simulink model "Admittance"  (R2022b)
settings: Solver=VariableStepAuto  StartTime=0.0  StopTime=10.0  RelTol=1e-3
values from neighbouring files (symbols this model uses):
  Kd = diag([10,10,10,1,1,1])    [parameters.m]
  Kdt = diag([5,5,5,1,1,1])    [parameters.m]
  Kp = diag([190,190,190,1,1,1])    [parameters.m]
  Kpt = diag([50,50,50,1,1,1])    [parameters.m]
  Md = diag([0.12,0.12,0.12,0,0,0])    [parameters.m]
  Mt = diag([1,1,1,1,1,1])    [parameters.m]
undefined symbols (not defined in the file or in its folder): parms
libraries: robotcorelib x1
settings Model: Creator=uzair  LastModifiedBy=uzair

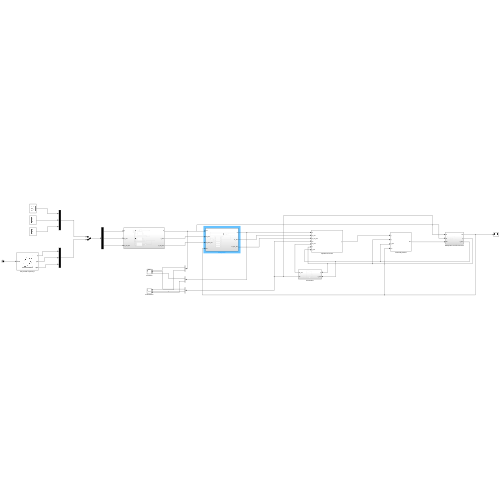
[thumbnail: Simulink's stored preview of the top-level diagram]
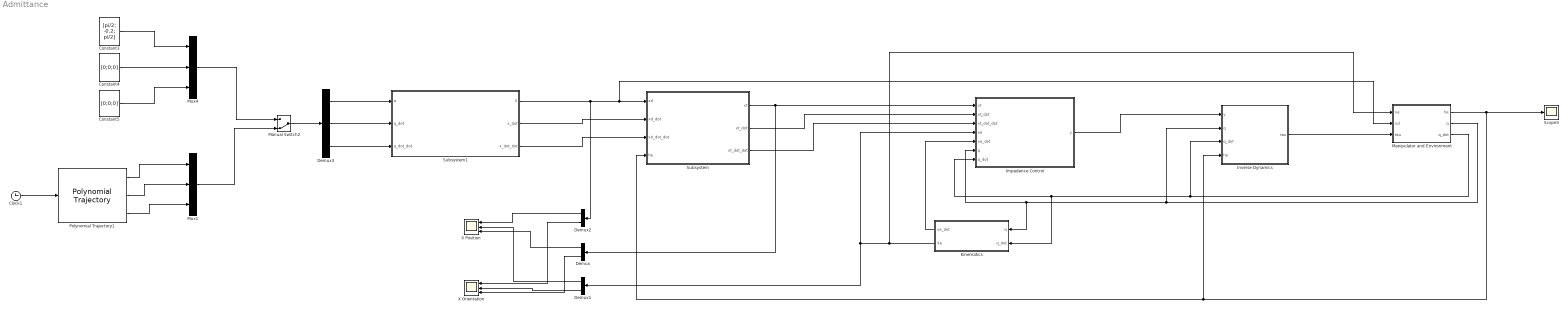
== system Admittance ==
  Clock1 : Clock
  Constant3 : Constant  Value=[pi/2; -0.2; pi/2]  VectorParams1D=off
  Constant4 : Constant  Value=[0;0;0]  VectorParams1D=off
  Constant5 : Constant  Value=[0;0;0]  VectorParams1D=off
  Demux : Demux  Outputs=2
  Demux1 : Demux  Outputs=2
  Demux2 : Demux  Outputs=2
  Demux3 : Demux  Outputs=3
  Impedence Control : Subsystem
  Inverse Dynamics : Subsystem
  Kinematics : Subsystem
  Manipulator and Environment : Subsystem
  Manual Switch2 : ManualSwitch  CurrentSetting=0
  Mux1 : Mux  Inputs=3
  Mux4 : Mux  Inputs=3
  Polynomial Trajectory1 : robotcorelib/Polynomial Trajectory  WaypointSource=Internal  Waypoints=[ 0,0.5,0.7,0.9; 0,-0.05,-0.1,-0.15; 0,0.5,0.7,0.9]  TimePoints=[ 0, 4, 7, 10]  TimeInterval=[ 1, 4 ]  Method=Quintic Polynomial  ParameterSource=Internal  VelocityBoundaryCondition=zeros( 3,4 )  AccelerationBoundaryCondition=zeros( 3,4 )  SimulateUsing=Interpreted execution
  Scope3 : Scope
  Subsystem : Subsystem
  Subsystem1 : Subsystem
  X Orientation : Scope  NumInputPorts=3
  X Position : Scope  NumInputPorts=3
  wires:
  Demux1/2 -> X Orientation/2
  Demux2/2 -> X Orientation/1
  Demux2/1 -> X Position/1
  Demux1/1 -> X Position/2
  Manual Switch2/1 -> Demux3/1
  Mux4/1 -> Manual Switch2/1
  Constant4/1 -> Mux4/2
  Polynomial Trajectory1/1 -> Mux1/1
  Polynomial Trajectory1/3 -> Mux1/3
  Mux1/1 -> Manual Switch2/2
  Constant5/1 -> Mux4/3
  Clock1/1 -> Polynomial Trajectory1/1
  Constant3/1 -> Mux4/1
  Demux3/3 -> Subsystem1/3(q_dot_dot)
  Polynomial Trajectory1/2 -> Mux1/2
  Demux3/2 -> Subsystem1/2(q_dot)
  Impedence Control/1(y) -> Inverse Dynamics/1(y)
  Kinematics/2(Xe) -> Manipulator and Environment/1(xe), Demux1/1, Impedence Control/4(xe)
  Kinematics/1(xe_dot) -> Impedence Control/5(xe_dot)
  Manipulator and Environment/2(q) -> Inverse Dynamics/2(q), Kinematics/1(q), Impedence Control/6(q)
  Manipulator and Environment/3(q_dot) -> Inverse Dynamics/3(q_dot), Kinematics/2(q_dot), Impedence Control/7(q_dot)
  Manipulator and Environment/1(he) -> Scope3/1, Inverse Dynamics/4(he), Subsystem/4(he)
  Inverse Dynamics/1(tau) -> Manipulator and Environment/3(tau)
  Demux3/1 -> Subsystem1/1(q)
  Subsystem1/1(X) -> Demux2/1, Manipulator and Environment/2(xd), Subsystem/1(xd)
  Subsystem1/2(x_dot) -> Subsystem/2(xd_dot)
  Subsystem1/3(x_dot_dot) -> Subsystem/3(xd_dot_dot)
  Subsystem/1(xt) -> Demux/1, Impedence Control/1(xt)
  Subsystem/2(xt_dot) -> Impedence Control/2(xt_dot)
  Subsystem/3(xt_dot_dot) -> Impedence Control/3(xt_dot_dot)
  Demux/1 -> X Position/3
  Demux/2 -> X Orientation/3

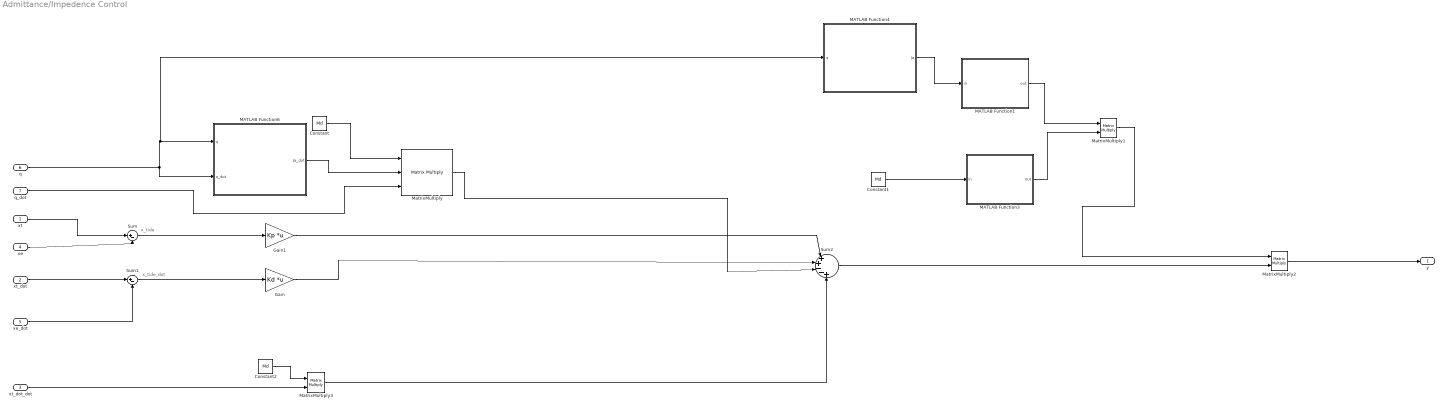
== system Admittance/Impedence Control ==
  note: x_tide_dot
  note: x_tide
  xt : Inport
  xt_dot : Inport  Port=2
  xt_dot_dot : Inport  Port=3
  xe : Inport  Port=4
  xe_dot : Inport  Port=5
  q : Inport  Port=6
  q_dot : Inport  Port=7
  Constant : Constant  Value=Md  VectorParams1D=off
  Constant1 : Constant  Value=Md  VectorParams1D=off
  Constant2 : Constant  Value=Md
  Gain : Gain  Gain=Kd  Multiplication=Matrix(K*u)
  Gain1 : Gain  Gain=Kp  Multiplication=Matrix(K*u)
  MATLAB Function1 : MATLAB Function  TreatAsAtomicUnit=on
  MATLAB Function3 : MATLAB Function  TreatAsAtomicUnit=on
  MATLAB Function4 : MATLAB Function  TreatAsAtomicUnit=on
  MATLAB Function6 : MATLAB Function  TreatAsAtomicUnit=on
  MatrixMultiply : Product  Inputs=3  Multiplication=Matrix(*)
  MatrixMultiply1 : Product  Multiplication=Matrix(*)
  MatrixMultiply2 : Product  Multiplication=Matrix(*)
  MatrixMultiply3 : Product  Multiplication=Matrix(*)
  Sum : Sum  Inputs=|+-
  Sum1 : Sum  Inputs=|+-
  Sum2 : Sum  Inputs=|++--+
  y : Outport
  wires:
  xt/1 -> Sum/1
  xe/1 -> Sum/2
  Sum/1 -> Gain1/1
  xt_dot/1 -> Sum1/1
  xe_dot/1 -> Sum1/2
  Sum1/1 -> Gain/1
  Gain1/1 -> Sum2/1
  Gain/1 -> Sum2/2
  q/1 -> MATLAB Function6/2(q_dot), MATLAB Function4/1(q), MATLAB Function6/1(q)
  q_dot/1 -> MatrixMultiply/3
  Constant/1 -> MatrixMultiply/1
  MATLAB Function6/1(Ja_dot) -> MatrixMultiply/2
  MatrixMultiply/1 -> Sum2/3
  MATLAB Function1/1(out) -> MatrixMultiply1/1
  MATLAB Function3/1(out) -> MatrixMultiply1/2
  MATLAB Function4/1(Ja) -> MATLAB Function1/1(in)
  Constant1/1 -> MATLAB Function3/1(in)
  Sum2/1 -> MatrixMultiply2/2
  MatrixMultiply1/1 -> MatrixMultiply2/1
  MatrixMultiply2/1 -> y/1
  xt_dot_dot/1 -> MatrixMultiply3/2
  Constant2/1 -> MatrixMultiply3/1
  MatrixMultiply3/1 -> Sum2/5

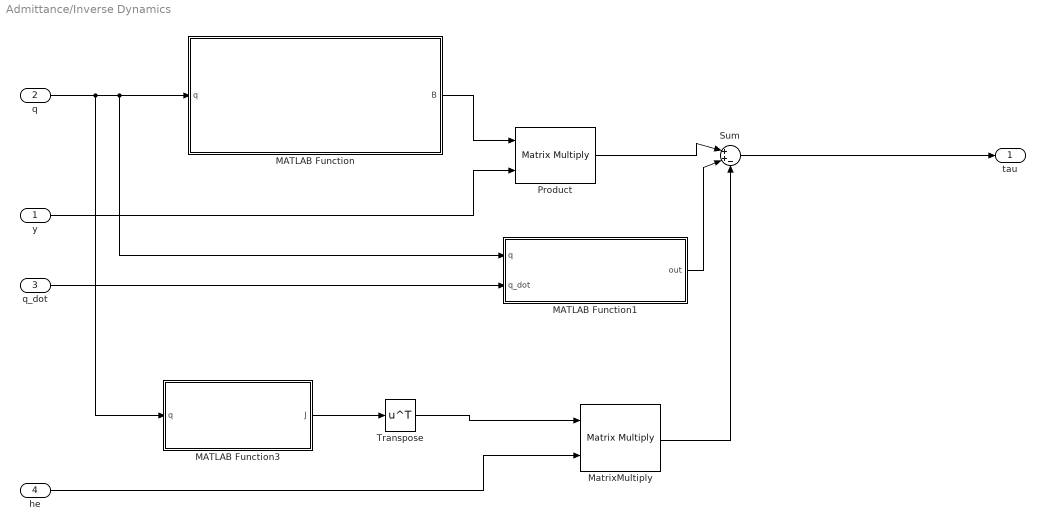
== system Admittance/Inverse Dynamics ==
  y : Inport
  q : Inport  Port=2
  q_dot : Inport  Port=3
  he : Inport  Port=4
  MATLAB Function : MATLAB Function  TreatAsAtomicUnit=on
  MATLAB Function1 : MATLAB Function  TreatAsAtomicUnit=on
  MATLAB Function3 : MATLAB Function  TreatAsAtomicUnit=on
  MatrixMultiply : Product  Multiplication=Matrix(*)
  Product : Product  Multiplication=Matrix(*)
  Sum : Sum  Inputs=|++-
  Transpose : Math  Operator=transpose  OutputSignalType=real
  tau : Outport
  wires:
  q/1 -> MATLAB Function3/1(q), MATLAB Function1/1(q), MATLAB Function/1(q)
  MATLAB Function/1(B) -> Product/1
  y/1 -> Product/2
  q_dot/1 -> MATLAB Function1/2(q_dot)
  MATLAB Function1/1(out) -> Sum/2
  Sum/1 -> tau/1
  MATLAB Function3/1(J) -> Transpose/1
  he/1 -> MatrixMultiply/2
  Transpose/1 -> MatrixMultiply/1
  MatrixMultiply/1 -> Sum/3
  Product/1 -> Sum/1

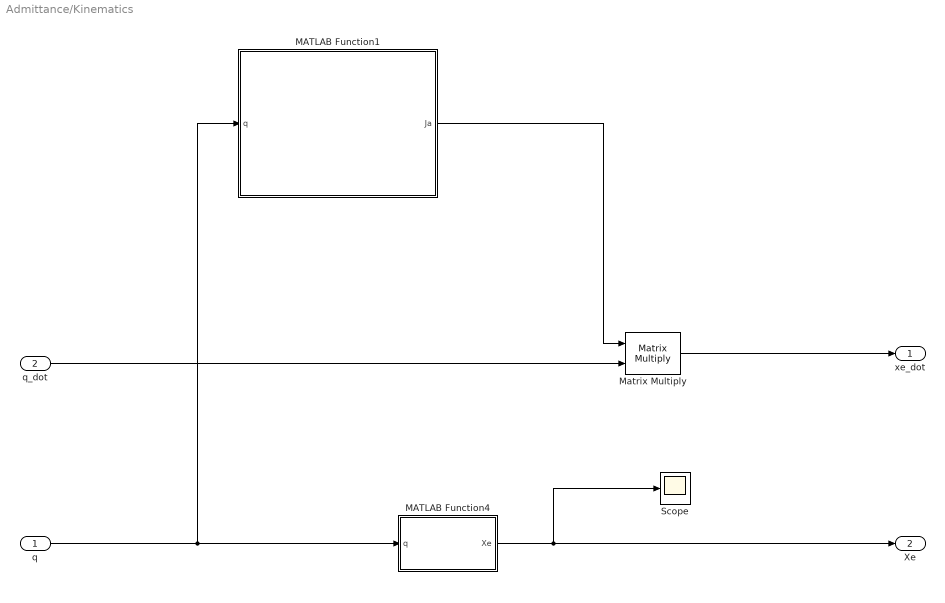
== system Admittance/Kinematics ==
  q : Inport
  q_dot : Inport  Port=2
  MATLAB Function1 : MATLAB Function  TreatAsAtomicUnit=on
  MATLAB Function4 : MATLAB Function  TreatAsAtomicUnit=on
  Matrix Multiply : Product  Multiplication=Matrix(*)
  Scope : Scope
  xe_dot : Outport
  Xe : Outport  Port=2
  wires:
  MATLAB Function1/1(Ja) -> Matrix Multiply/1
  q/1 -> MATLAB Function1/1(q), MATLAB Function4/1(q)
  MATLAB Function4/1(Xe) -> Scope/1, Xe/1
  Matrix Multiply/1 -> xe_dot/1
  q_dot/1 -> Matrix Multiply/2

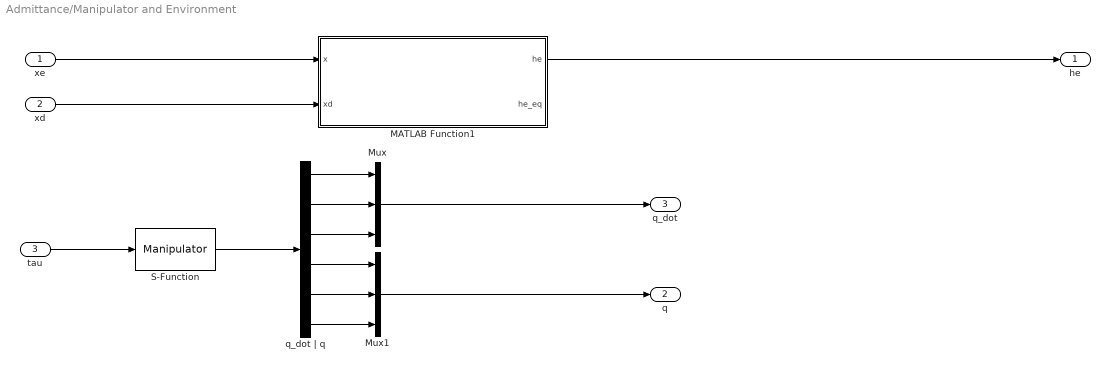
== system Admittance/Manipulator and Environment ==
  xe : Inport
  xd : Inport  Port=2
  tau : Inport  Port=3
  MATLAB Function1 : MATLAB Function  TreatAsAtomicUnit=on
  Mux : Mux  Inputs=3
  Mux1 : Mux  Inputs=3
  S-Function : S-Function  FunctionName=Manipulator  Parameters=params  SFunctionDeploymentMode=off  EnableBusSupport=off
  q_dot | q : Demux  Outputs=6
  he : Outport
  q : Outport  Port=2
  q_dot : Outport  Port=3
  wires:
  xe/1 -> MATLAB Function1/1(x)
  xd/1 -> MATLAB Function1/2(xd)
  MATLAB Function1/1(he) -> he/1
  S-Function/1 -> q_dot | q/1
  q_dot | q/4 -> Mux1/1
  q_dot | q/1 -> Mux/1
  q_dot | q/6 -> Mux1/3
  q_dot | q/2 -> Mux/2
  q_dot | q/5 -> Mux1/2
  q_dot | q/3 -> Mux/3
  Mux/1 -> q_dot/1
  Mux1/1 -> q/1
  tau/1 -> S-Function/1

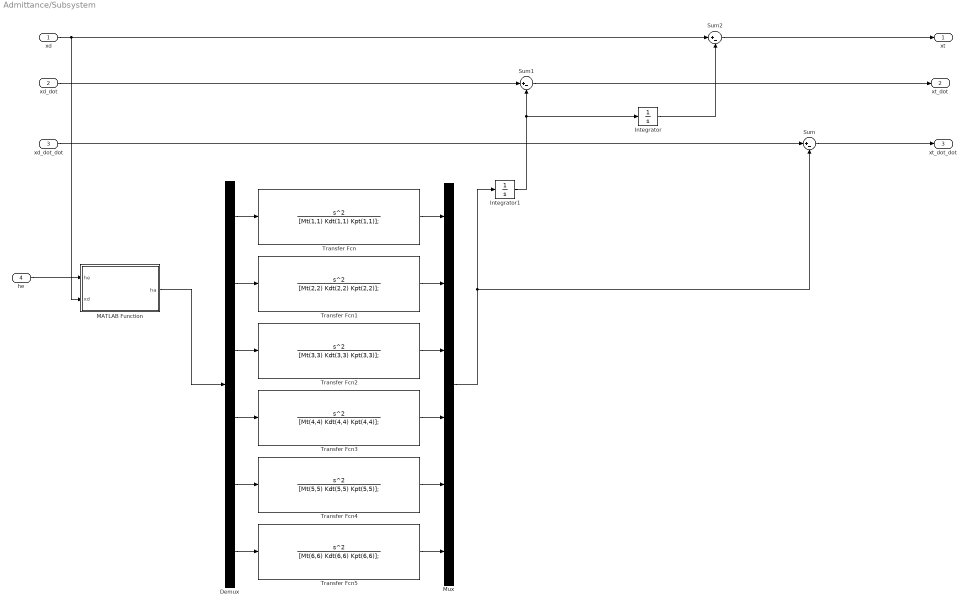
== system Admittance/Subsystem ==
  xd : Inport
  xd_dot : Inport  Port=2
  xd_dot_dot : Inport  Port=3
  he : Inport  Port=4
  Demux : Demux  Outputs=6
  Integrator : Integrator
  Integrator1 : Integrator
  MATLAB Function : MATLAB Function  TreatAsAtomicUnit=on
  Mux : Mux  Inputs=6
  Sum : Sum  Inputs=|+-
  Sum1 : Sum  Inputs=|+-
  Sum2 : Sum  Inputs=|+-
  Transfer Fcn : TransferFcn  Numerator=[1 0 0]  Denominator=[Mt(1,1) Kdt(1,1) Kpt(1,1)];
  Transfer Fcn1 : TransferFcn  Numerator=[1 0 0]  Denominator=[Mt(2,2) Kdt(2,2) Kpt(2,2)];
  Transfer Fcn2 : TransferFcn  Numerator=[1 0 0]  Denominator=[Mt(3,3) Kdt(3,3) Kpt(3,3)];
  Transfer Fcn3 : TransferFcn  Numerator=[1 0 0]  Denominator=[Mt(4,4) Kdt(4,4) Kpt(4,4)];
  Transfer Fcn4 : TransferFcn  Numerator=[1 0 0]  Denominator=[Mt(5,5) Kdt(5,5) Kpt(5,5)];
  Transfer Fcn5 : TransferFcn  Numerator=[1 0 0]  Denominator=[Mt(6,6) Kdt(6,6) Kpt(6,6)];
  xt : Outport
  xt_dot : Outport  Port=2
  xt_dot_dot : Outport  Port=3
  wires:
  he/1 -> MATLAB Function/1(he)
  xd/1 -> Sum2/1, MATLAB Function/2(xd)
  Sum2/1 -> xt/1
  xd_dot/1 -> Sum1/1
  Sum1/1 -> xt_dot/1
  Sum/1 -> xt_dot_dot/1
  xd_dot_dot/1 -> Sum/1
  MATLAB Function/1(ha) -> Demux/1
  Mux/1 -> Integrator1/1, Sum/2
  Integrator1/1 -> Integrator/1, Sum1/2
  Integrator/1 -> Sum2/2
  Transfer Fcn/1 -> Mux/1
  Demux/1 -> Transfer Fcn/1
  Demux/2 -> Transfer Fcn1/1
  Transfer Fcn1/1 -> Mux/2
  Demux/3 -> Transfer Fcn2/1
  Transfer Fcn2/1 -> Mux/3
  Transfer Fcn3/1 -> Mux/4
  Demux/4 -> Transfer Fcn3/1
  Transfer Fcn4/1 -> Mux/5
  Demux/5 -> Transfer Fcn4/1
  Transfer Fcn5/1 -> Mux/6
  Demux/6 -> Transfer Fcn5/1

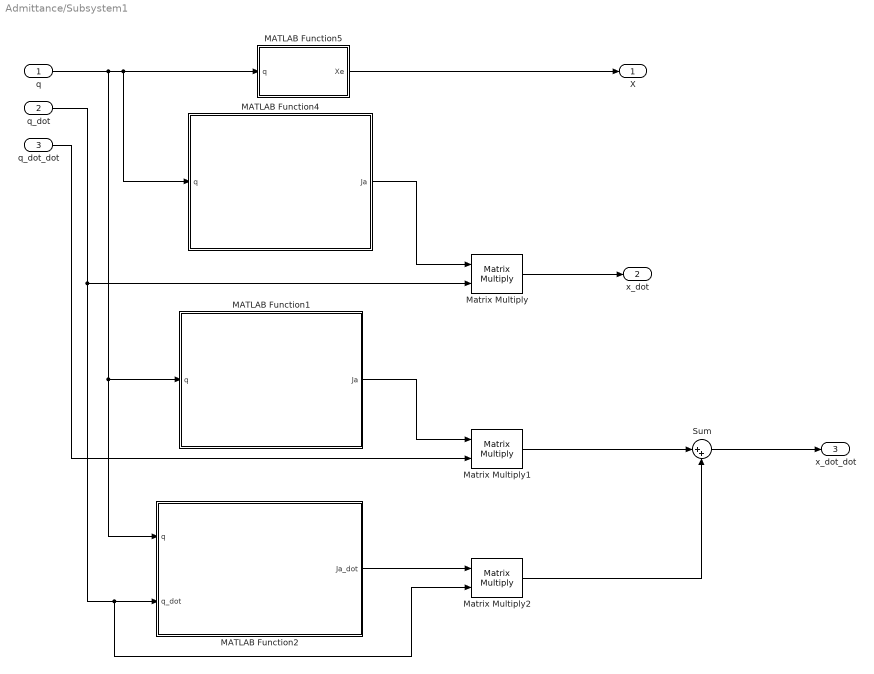
== system Admittance/Subsystem1 ==
  q : Inport
  q_dot : Inport  Port=2
  q_dot_dot : Inport  Port=3
  MATLAB Function1 : MATLAB Function  TreatAsAtomicUnit=on
  MATLAB Function2 : MATLAB Function  TreatAsAtomicUnit=on
  MATLAB Function4 : MATLAB Function  TreatAsAtomicUnit=on
  MATLAB Function5 : MATLAB Function  TreatAsAtomicUnit=on
  Matrix Multiply : Product  Multiplication=Matrix(*)
  Matrix Multiply1 : Product  Multiplication=Matrix(*)  SaturateOnIntegerOverflow=on  LockScale=on
  Matrix Multiply2 : Product  Multiplication=Matrix(*)  InputSameDT=on  SaturateOnIntegerOverflow=on
  Sum : Sum  Inputs=|++
  X : Outport
  x_dot : Outport  Port=2
  x_dot_dot : Outport  Port=3
  wires:
  q/1 -> MATLAB Function2/1(q), MATLAB Function1/1(q), MATLAB Function4/1(q), MATLAB Function5/1(q)
  MATLAB Function5/1(Xe) -> X/1
  Matrix Multiply/1 -> x_dot/1
  q_dot/1 -> MATLAB Function2/2(q_dot), Matrix Multiply2/2, Matrix Multiply/2
  MATLAB Function4/1(Ja) -> Matrix Multiply/1
  MATLAB Function1/1(Ja) -> Matrix Multiply1/1
  q_dot_dot/1 -> Matrix Multiply1/2
  Matrix Multiply1/1 -> Sum/1
  Sum/1 -> x_dot_dot/1
  MATLAB Function2/1(Ja_dot) -> Matrix Multiply2/1
  Matrix Multiply2/1 -> Sum/2

== matlab function Admittance/Impedence Control/MATLAB Function6 ==
  data: q input; Ja_dot output; q_dot input
function Ja_dot = AnalyticalJacobian_Dot(q, q_dot)
q1 = q(1);
q2 = q(2);
q3 = q(3);

q1_dot = q_dot(1);
q2_dot = q_dot(2);
q3_dot = q_dot(3);

H = [[       0,         -cos(q3),        -sin(q3),                                                     -(4*sin(q3))/25]
[ sin(q1), -cos(q1)*sin(q3), cos(q1)*cos(q3),        (2*cos(q1))/5 + (4*cos(q1)*cos(q3))/25 - sin(q1)*(q2 + 3/10)]
[-cos(q1), -sin(q1)*sin(q3), cos(q3)*sin(q1), (2*sin(q1))/5 + cos(q1)*(q2 + 3/10) + (4*cos(q3)*sin(q1))/25 + 3/20]
[       0,                0,               0,                                                                   1]];



eulers = rotm2eul(H(1:3,1:3), "ZYZ");


phi1 = eulers(1);
phi2 = eulers(2);
phi3 = eulers(3); %not used

Ja_dot_m = [
[                                                                                                                                   0,               0,                                                 (4*q3_dot*sin(q3))/25]
[  q1_dot*sin(q1)*(q2 + 3/10) - q2_dot*cos(q1) - (4*q1_dot*cos(q1)*cos(q3))/25 - (2*q1_dot*cos(q1))/5 + (4*q3_dot*sin(q1)*sin(q3))/25, -q1_dot*cos(q1),         (4*q1_dot*sin(q1)*sin(q3))/25 - (4*q3_dot*cos(q1)*cos(q3))/25]
[- (2*q1_dot*sin(q1))/5 - q2_dot*sin(q1) - q1_dot*cos(q1)*(q2 + 3/10) - (4*q1_dot*cos(q3)*sin(q1))/25 - (4*q3_dot*cos(q1)*sin(q3))/25, -q1_dot*sin(q1),       - (4*q1_dot*cos(q1)*sin(q3))/25 - (4*q3_dot*cos(q3)*sin(q1))/25]
[                                                                                                                                   0,               0, -(q1_dot*(sin(phi2)*sin(q1) - cos(phi2)*cos(q1)*sin(phi1)))/sin(phi2)]
[                                                                                                                                   0,               0,                                             -q1_dot*cos(phi1)*cos(q1)]
[                                                                                                                                   0,               0,                                 -(q1_dot*cos(q1)*sin(phi1))/sin(phi2)]
];

Ja_dot = Ja_dot_m;
end

== matlab function Admittance/Subsystem1/MATLAB Function2 ==
  data: q input; Ja_dot output; q_dot input
function Ja_dot = AnalyticalJacobian_Dot(q, q_dot)
q1 = q(1);
q2 = q(2);
q3 = q(3);

q1_dot = q_dot(1);
q2_dot = q_dot(2);
q3_dot = q_dot(3);

H = [[       0,         -cos(q3),        -sin(q3),                                                     -(4*sin(q3))/25]
[ sin(q1), -cos(q1)*sin(q3), cos(q1)*cos(q3),        (2*cos(q1))/5 + (4*cos(q1)*cos(q3))/25 - sin(q1)*(q2 + 3/10)]
[-cos(q1), -sin(q1)*sin(q3), cos(q3)*sin(q1), (2*sin(q1))/5 + cos(q1)*(q2 + 3/10) + (4*cos(q3)*sin(q1))/25 + 3/20]
[       0,                0,               0,                                                                   1]];



eulers = rotm2eul(H(1:3,1:3), "ZYZ");


phi1 = eulers(1);
phi2 = eulers(2);
phi3 = eulers(3); %not used

Ja_dot_m = [
[                                                                                                                                   0,               0,                                                 (4*q3_dot*sin(q3))/25]
[  q1_dot*sin(q1)*(q2 + 3/10) - q2_dot*cos(q1) - (4*q1_dot*cos(q1)*cos(q3))/25 - (2*q1_dot*cos(q1))/5 + (4*q3_dot*sin(q1)*sin(q3))/25, -q1_dot*cos(q1),         (4*q1_dot*sin(q1)*sin(q3))/25 - (4*q3_dot*cos(q1)*cos(q3))/25]
[- (2*q1_dot*sin(q1))/5 - q2_dot*sin(q1) - q1_dot*cos(q1)*(q2 + 3/10) - (4*q1_dot*cos(q3)*sin(q1))/25 - (4*q3_dot*cos(q1)*sin(q3))/25, -q1_dot*sin(q1),       - (4*q1_dot*cos(q1)*sin(q3))/25 - (4*q3_dot*cos(q3)*sin(q1))/25]
[                                                                                                                                   0,               0, -(q1_dot*(sin(phi2)*sin(q1) - cos(phi2)*cos(q1)*sin(phi1)))/sin(phi2)]
[                                                                                                                                   0,               0,                                             -q1_dot*cos(phi1)*cos(q1)]
[                                                                                                                                   0,               0,                                 -(q1_dot*cos(q1)*sin(phi1))/sin(phi2)]
];

Ja_dot = Ja_dot_m;
end

== matlab function Admittance/Subsystem1/MATLAB Function4 ==
  data: q input; Ja output
function Ja = AnalyticalJacobian(q)
    q1 = q(1);
    q2 = q(2);
    q3 = q(3);

    H = [[       0,         -cos(q3),        -sin(q3),                                                     -(4*sin(q3))/25]
[ sin(q1), -cos(q1)*sin(q3), cos(q1)*cos(q3),        (2*cos(q1))/5 + (4*cos(q1)*cos(q3))/25 - sin(q1)*(q2 + 3/10)]
[-cos(q1), -sin(q1)*sin(q3), cos(q3)*sin(q1), (2*sin(q1))/5 + cos(q1)*(q2 + 3/10) + (4*cos(q3)*sin(q1))/25 + 3/20]
[       0,                0,               0,                                                                   1]];


eulers = rotm2eul(H(1:3,1:3), "ZYZ");


    phi1 = eulers(1);
    phi2 = eulers(2);
    phi3 = eulers(3); %not used

Ja_m = [
[                                                             0,        0,                                             -(4*cos(q3))/25]
[- (2*sin(q1))/5 - cos(q1)*(q2 + 3/10) - (4*cos(q3)*sin(q1))/25, -sin(q1),                                     -(4*cos(q1)*sin(q3))/25]
[  (2*cos(q1))/5 + (4*cos(q1)*cos(q3))/25 - sin(q1)*(q2 + 3/10),  cos(q1),                                     -(4*sin(q1)*sin(q3))/25]
[                              -(cos(phi1)*cos(phi2))/sin(phi2),        0, (cos(q1)*sin(phi2) + cos(phi2)*sin(phi1)*sin(q1))/sin(phi2)]
[                                                    -sin(phi1),        0,                                          -cos(phi1)*sin(q1)]
[                                           cos(phi1)/sin(phi2),        0,                              -(sin(phi1)*sin(q1))/sin(phi2)]
];


    Ja = Ja_m;
end

== matlab function Admittance/Subsystem1/MATLAB Function5 ==
  data: q input; Xe output
function Xe = Kinematics(q)
    q1 = q(1);
    q2 = q(2);
    q3 = q(3);
    
H = [[       0,         -cos(q3),        -sin(q3),                                                     -(4*sin(q3))/25]
[ sin(q1), -cos(q1)*sin(q3), cos(q1)*cos(q3),        (2*cos(q1))/5 + (4*cos(q1)*cos(q3))/25 - sin(q1)*(q2 + 3/10)]
[-cos(q1), -sin(q1)*sin(q3), cos(q3)*sin(q1), (2*sin(q1))/5 + cos(q1)*(q2 + 3/10) + (4*cos(q3)*sin(q1))/25 + 3/20]
[       0,                0,               0,                                                                   1]];


    eulers = rotm2eul(H(1:3,1:3), "ZYZ");

    Xe = [H(1:3,4); eulers'];
end

== matlab function Admittance/Inverse Dynamics/MATLAB Function1 ==
  data: q input; out output; q_dot input; params parameter
function out = n(q, q_dot, params)
    
    m1 = params.m(1);
    m2 = params.m(2);
    m3 = params.m(3);

    q1 = q(1);
    q2 = q(2);
    q3 = q(3);

    q1_dot = q_dot(1);
    q2_dot = q_dot(2);
    q3_dot = q_dot(3);

    g = params.g;

    Fv = params.Fv;
 

    C = [[q2_dot*((3*m2)/20 + (3*m3)/10 + m2*q2 + m3*q2) - q3_dot*((4*m3*sin(2*q3))/625 + (4*m3*sin(q3))/125), q1_dot*((3*m2)/20 + (3*m3)/10 + m2*q2 + m3*q2), (2*m3*q3_dot*cos(q3)*(q2 + 3/10))/25 - q1_dot*((4*m3*sin(q3))/125 + (8*m3*cos(q3)*sin(q3))/625)]
        [                        -q1_dot*((3*m2)/20 + (3*m3)/10 + m2*q2 + m3*q2) - (2*m3*q3_dot*sin(q3))/25,                                              0,                                                                       -(2*m3*q1_dot*sin(q3))/25]
        [                      q1_dot*((4*m3*sin(2*q3))/625 + (4*m3*sin(q3))/125) + (2*m3*q2_dot*sin(q3))/25,                       (2*m3*q1_dot*sin(q3))/25,                                                                                               0]];

    G = [(g*m1*cos(q1))/5 - g*m2*((3*sin(q1))/20 - (2*cos(q1))/5 + q2*sin(q1)) + g*m3*((2*cos(q1))/5 + (2*cos(q1)*cos(q3))/25 - sin(q1)*(q2 + 3/10));
                                                                                                                        g*cos(q1)*(m2 + m3);
                                                                                                               -(2*g*m3*sin(q1)*sin(q3))/25];

    out = C*q_dot + diag(Fv)*q_dot + G;
end

== matlab function Admittance/Inverse Dynamics/MATLAB Function ==
  data: q input; B output; params parameter
function B = inertiaMatrix(q, params)
    q1 = q(1); % not used in this matrix
    q2 = q(2);
    q3 = q(3);

    m1 = params.m(1);
    m2 = params.m(2);
    m3 = params.m(3);

    B = [[(195791581307*m1)/1220703125000 + (8503*m2)/40000 + (321279862557*m3)/1220703125000 + (8*m3*cos(q3)^2)/625 + (3*m2*q2)/10 + (3*m3*q2)/5 + m2*q2^2 + m3*q2^2 + (8*m3*cos(q3))/125, (2*m2)/5 + (2*m3)/5 + (2*m3*cos(q3))/25, (2*m3*sin(q3)*(q2 + 3/10))/25]
        [                                                                                                                                         (2*m2)/5 + (2*m3)/5 + (2*m3*cos(q3))/25,                                 m2 + m3,                             0]
        [                                                                                                                                                   (2*m3*sin(q3)*(q2 + 3/10))/25,                                       0,            (32637*m3)/1562500]];
end

== matlab function Admittance/Subsystem1/MATLAB Function1 ==
  data: q input; Ja output
function Ja = AnalyticalJacobian(q)
    q1 = q(1);
    q2 = q(2);
    q3 = q(3);

    H = [[       0,         -cos(q3),        -sin(q3),                                                     -(4*sin(q3))/25]
[ sin(q1), -cos(q1)*sin(q3), cos(q1)*cos(q3),        (2*cos(q1))/5 + (4*cos(q1)*cos(q3))/25 - sin(q1)*(q2 + 3/10)]
[-cos(q1), -sin(q1)*sin(q3), cos(q3)*sin(q1), (2*sin(q1))/5 + cos(q1)*(q2 + 3/10) + (4*cos(q3)*sin(q1))/25 + 3/20]
[       0,                0,               0,                                                                   1]];


eulers = rotm2eul(H(1:3,1:3), "ZYZ");


    phi1 = eulers(1);
    phi2 = eulers(2);
    phi3 = eulers(3); %not used

Ja_m = [
[                                                             0,        0,                                             -(4*cos(q3))/25]
[- (2*sin(q1))/5 - cos(q1)*(q2 + 3/10) - (4*cos(q3)*sin(q1))/25, -sin(q1),                                     -(4*cos(q1)*sin(q3))/25]
[  (2*cos(q1))/5 + (4*cos(q1)*cos(q3))/25 - sin(q1)*(q2 + 3/10),  cos(q1),                                     -(4*sin(q1)*sin(q3))/25]
[                              -(cos(phi1)*cos(phi2))/sin(phi2),        0, (cos(q1)*sin(phi2) + cos(phi2)*sin(phi1)*sin(q1))/sin(phi2)]
[                                                    -sin(phi1),        0,                                          -cos(phi1)*sin(q1)]
[                                           cos(phi1)/sin(phi2),        0,                              -(sin(phi1)*sin(q1))/sin(phi2)]
];


    Ja = Ja_m;
end

== matlab function Admittance/Subsystem/MATLAB Function ==
  data: he input; ha output; xd input
function ha = he_d_e(he, xd)

        euler = xd(4:6);

        phi1 = euler(1);
        phi2 = euler(2);

        T = [[0, -sin(phi1) ,    cos(phi1)*sin(phi2)];
                 [0,  cos(phi1) ,   sin(phi1)*sin(phi2)];
                 [1,               0  ,    cos(phi2)]];

        Ta = [[eye(3), zeros(3)];
              [zeros(3), T]];


        ha = Ta'*he;
end

== matlab function Admittance/Kinematics/MATLAB Function4 ==
  data: q input; Xe output
function Xe = Kinematics(q)
    q1 = q(1);
    q2 = q(2);
    q3 = q(3);
    
    H = [[       0,         -cos(q3),        -sin(q3),                                                     -(4*sin(q3))/25]
         [ sin(q1), -cos(q1)*sin(q3), cos(q1)*cos(q3),        (2*cos(q1))/5 + (4*cos(q1)*cos(q3))/25 - sin(q1)*(q2 + 3/10)]
         [-cos(q1), -sin(q1)*sin(q3), cos(q3)*sin(q1), (2*sin(q1))/5 + cos(q1)*(q2 + 3/10) + (4*cos(q3)*sin(q1))/25 + 3/20]
         [       0,                0,               0,                                                                   1]];


    eulers = rotm2eul(H(1:3,1:3), "ZYZ");

    Xe = [H(1:3,4); eulers'];
end

== matlab function Admittance/Impedence Control/MATLAB Function1 ==
  data: in input; out output
function out = inv(in)
    out = pinv(in);
end

== matlab function Admittance/Kinematics/MATLAB Function1 ==
  data: q input; Ja output
function Ja = AnalyticalJacobian(q)
    q1 = q(1);
    q2 = q(2);
    q3 = q(3);

    H = [[       0,         -cos(q3),        -sin(q3),                                                     -(4*sin(q3))/25]
[ sin(q1), -cos(q1)*sin(q3), cos(q1)*cos(q3),        (2*cos(q1))/5 + (4*cos(q1)*cos(q3))/25 - sin(q1)*(q2 + 3/10)]
[-cos(q1), -sin(q1)*sin(q3), cos(q3)*sin(q1), (2*sin(q1))/5 + cos(q1)*(q2 + 3/10) + (4*cos(q3)*sin(q1))/25 + 3/20]
[       0,                0,               0,                                                                   1]];


eulers = rotm2eul(H(1:3,1:3), "ZYZ");


    phi1 = eulers(1);
    phi2 = eulers(2);
    phi3 = eulers(3); %not used

Ja_m = [
[                                                             0,        0,                                             -(4*cos(q3))/25]
[- (2*sin(q1))/5 - cos(q1)*(q2 + 3/10) - (4*cos(q3)*sin(q1))/25, -sin(q1),                                     -(4*cos(q1)*sin(q3))/25]
[  (2*cos(q1))/5 + (4*cos(q1)*cos(q3))/25 - sin(q1)*(q2 + 3/10),  cos(q1),                                     -(4*sin(q1)*sin(q3))/25]
[                              -(cos(phi1)*cos(phi2))/sin(phi2),        0, (cos(q1)*sin(phi2) + cos(phi2)*sin(phi1)*sin(q1))/sin(phi2)]
[                                                    -sin(phi1),        0,                                          -cos(phi1)*sin(q1)]
[                                           cos(phi1)/sin(phi2),        0,                              -(sin(phi1)*sin(q1))/sin(phi2)]
];


    Ja = Ja_m;
end

== matlab function Admittance/Manipulator and Environment/MATLAB Function1 ==
  data: x input; he output; xd input; parms parameter; Kp parameter; he_eq output
function [he,he_eq]= Environment(x, xd, parms, Kp)
    if(x(parms.plane_axis) >= parms.plane_pos(parms.plane_axis))
        xr = parms.plane_pos;

        xdes = zeros(6,1);
        xdes(parms.plane_axis) = xd(parms.plane_axis);

        xe = zeros(6,1);
        xe(parms.plane_axis) = x(parms.plane_axis);

        he = parms.Ke * (xe - xr);

        he_eq = pinv(eye(6) + parms.Ke*pinv(Kp))*parms.Ke*(xdes - xr);

    else
        he = zeros(6,1);
        he_eq = zeros(6,1);
    end
end

== matlab function Admittance/Impedence Control/MATLAB Function3 ==
  data: in input; out output
function out = inv(in)
    out = pinv(in);
end

== matlab function Admittance/Impedence Control/MATLAB Function4 ==
  data: q input; Ja output
function Ja = AnalyticalJacobian(q)
    
    q1 = q(1);
    q2 = q(2);
    q3 = q(3);

       H = [[       0,         -cos(q3),        -sin(q3),                                                     -(4*sin(q3))/25]
         [ sin(q1), -cos(q1)*sin(q3), cos(q1)*cos(q3),        (2*cos(q1))/5 + (4*cos(q1)*cos(q3))/25 - sin(q1)*(q2 + 3/10)]
         [-cos(q1), -sin(q1)*sin(q3), cos(q3)*sin(q1), (2*sin(q1))/5 + cos(q1)*(q2 + 3/10) + (4*cos(q3)*sin(q1))/25 + 3/20]
         [       0,                0,               0,                                                                   1]];


        eulers = rotm2eul(H(1:3,1:3), "ZYZ");


        phi1 = eulers(1);
        phi2 = eulers(2);
        phi3 = eulers(3); %not used

        Ja = [
               [                                                                     0,        0,                                             -(4*cos(q3))/25]
               [- (3*cos(q1))/10 - (2*sin(q1))/5 - (4*cos(q3)*sin(q1))/25 - q2*cos(q1), -sin(q1),                                     -(4*cos(q1)*sin(q3))/25]
               [  (2*cos(q1))/5 - (3*sin(q1))/10 + (4*cos(q1)*cos(q3))/25 - q2*sin(q1),  cos(q1),                                     -(4*sin(q1)*sin(q3))/25]
               [                                      -(cos(phi1)*cos(phi2))/sin(phi2),        0, (cos(q1)*sin(phi2) + cos(phi2)*sin(phi1)*sin(q1))/sin(phi2)]
               [                                                            -sin(phi1),        0,                                          -cos(phi1)*sin(q1)]
               [                                                   cos(phi1)/sin(phi2),        0,                              -(sin(phi1)*sin(q1))/sin(phi2)]];

end

== matlab function Admittance/Inverse Dynamics/MATLAB Function3 ==
  data: q input; J output
function J = GeomatricalJacobian(q)
q1 = q(1);
q2 = q(2);
q3 = q(3);

    J = [
[                                                             0,        0,         -(4*cos(q3))/25]
[- (2*sin(q1))/5 - cos(q1)*(q2 + 3/10) - (4*cos(q3)*sin(q1))/25, -sin(q1), -(4*cos(q1)*sin(q3))/25]
[  (2*cos(q1))/5 + (4*cos(q1)*cos(q3))/25 - sin(q1)*(q2 + 3/10),  cos(q1), -(4*sin(q1)*sin(q3))/25]
[                                                             1,        0,                       0]
[                                                            0,        0,                -sin(q1)]
[                                                             0,        0,                 cos(q1)]];

end
